simulink model "craig_control"  (R2016a)
settings: Solver=VariableStepAuto  StartTime=0.0  StopTime=tray_time  FixedStep=time_per_step  MaxStep=0.005  RelTol=1e-3
undefined symbols (not defined in the file): jacob0, kp, kv, my_inv_j, robot_model
libraries: roblocks x5, vector_sweep x2
settings Model: ExtModeTrigMode=oneshot  ExtModeArmWhenConnect=off  Creator=pic  LastModifiedBy=Nahuel
settings SolverCC: ZeroCrossControl=DisableAll
settings DataIOCC: SaveFormat=Array  SignalLoggingSaveFormat=ModelDataLogs  ReturnWorkspaceOutputs=on
settings OptimizationCC: BlockReduction=off  BooleanDataType=off  ExpressionDepthLimit=2147483647  InitFltsAndDblsToZero=on
settings DebuggingCC: SaveWithParameterizedLinksMsg=none  UnderspecifiedInitializationDetection=Classic  MergeDetectMultiDrivingBlocksExec=none  SignalResolutionControl=TryResolveAllWithWarning  MultiTaskDSMMsg=warning  MultiTaskCondExecSysMsg=none  FcnCallInpInsideContextMsg=UseLocalSettings  StateNameClashWarn=warning
settings HardwareCC: ProdBitPerPointer=32  ProdLargestAtomicFloat=None  ProdIntDivRoundTo=Undefined  ProdEndianess=Unspecified  ProdWordSize=32  ProdHWDeviceType=32-bit Generic  TargetUnknown=on
settings ModelReferenceCC: PropagateSignalLabelsOutOfModel=off
settings GRTTargetCC: ModelReferenceCompliant=off  CompOptLevelCompliant=off  CombineOutputUpdateFcns=off  MatFileLogging=off  GRTInterface=on
settings ConfigComp: CovModelRefEnable=Off

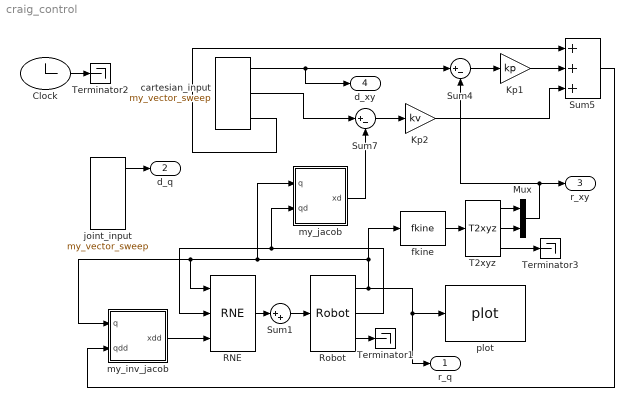
== system craig_control ==
  Clock : Clock
  Kp1 : Gain  Gain=kp  SaturateOnIntegerOverflow=on  OutDataTypeStr=Inherit: Same as input  ParamDataTypeStr=Inherit: Same as input
  Kp2 : Gain  Gain=kv  SaturateOnIntegerOverflow=on  OutDataTypeStr=Inherit: Same as input  ParamDataTypeStr=Inherit: Same as input
  Mux : Mux  Inputs=2
  RNE : roblocks/Dynamics/RNE  robot=robot_model  grav=[0 0 9.81]
  Robot : roblocks/Dynamics/Robot  robot=robot_real  q0=[-pi/2 pi/2]
  Sum1 : Sum  Inputs=|++  SaturateOnIntegerOverflow=on  InputSameDT=on  OutDataTypeStr=Inherit: Same as first input
  Sum4 : Sum  Inputs=|+-  SaturateOnIntegerOverflow=on  InputSameDT=on  OutDataTypeStr=Inherit: Same as first input
  Sum5 : Sum  Inputs=+++  SaturateOnIntegerOverflow=on  InputSameDT=on  OutDataTypeStr=Inherit: Same as first input
  Sum7 : Sum  Inputs=|+-  SaturateOnIntegerOverflow=on  InputSameDT=on  OutDataTypeStr=Inherit: Same as first input
  T2xyz : roblocks/Transform Conversion/T2xyz
  Terminator1 : Terminator
  Terminator2 : Terminator
  Terminator3 : Terminator
  cartesian_input : vector_sweep/my_vector_sweep  q_in=x_in  qd_in=xd_in  qdd_in=qdd_in  tmax=tray_time
  fkine : roblocks/Kinematics/fkine  robot=robot_model
  joint_input : vector_sweep/my_vector_sweep  q_in=q_in  qd_in=qd_in  qdd_in=qdd_in  tmax=tray_time
  my_inv_jacob : Subsystem  AncestorBlock=vector_sweep/my_inv_jacob
      mask help: Inverse Jacobian
      mask Help:
      | Inverse of Jacobian matrix which maps spatial velocity to joint coordinate
      | rates.
      | 
      | 
      | <b>Inputs::</b>
      | 
      | J (6x6) the Jacobian matrix
      | 
      | <b>Outputs::</b>
      | 
      | Ji (6x6) the inverse Jacobian matrix
      | 
      | <b>Notes::</b>
      | 
      | - A wrapper for the MATLAB function inv().
      | - Only valid for square Jacobians (6-axis robots)
      mask Display:
      | text(0.4, 0.7, '\bf\fontsize{16}J', 'texmode', 'on', 'verticalAlignment', 'top', 'horizontalAlignment', 'left')
      | text(0.6, 0.65, '\fontsize{10}-1', 'texmode', 'on','verticalAlignment', 'bottom', 'horizontalAlignment', 'left')
      | port_label('input', 1, 'q');
      | port_label('input', 2, 'xdd');
      | port_label('output', 1, 'qdd');
  "my_jacob " : Subsystem  AncestorBlock=vector_sweep/my_jacob  mask{robot=robot_model}
      mask prompts: robot "Robot object"
      mask help: Robot Jacobian in world coordinates
      mask init:
      | n=robot.n;
      mask Help:
      | Jacobian matrix relating joint coordinate rates to end-effector spatial
      | velocity expressed in the world frame.
      | 
      | <b>Parameters::</b>
      | 
      | Robot (SerialLink class)  The N-axis robot object for which the Jacobian is
      |                           computed.
      | 
      | <b>Inputs::</b>
      | 
      | q (1xN) joint coordinates
      | 
      | <b>Outputs::</b>
      | 
      | J (6xN) the Jacobian matrix
      | 
      | <b>Notes::</b>
      | 
      | - A wrapper for the Toolbox method jacob0().
      mask Display:
      | text(0.4, 0.7, '\bf\fontsize{16}J', 'texmode', 'on', 'verticalAlignment', 'top', 'horizontalAlignment', 'left')
      | text(0.45, 0.65, '\fontsize{10}0', 'texmode', 'on','verticalAlignment', 'bottom', 'horizontalAlignment', 'right')
      | if ~isempty(robot)
      |     text(0.5, 0.2, robot.name,  'horizontalAlignment', 'center')
      | end
      | port_label('input', 1, 'q')
      | port_label('input', 2, 'qd')
      | port_label('output', 1, 'xd')
  plot : roblocks/Robot Graphics/plot  robot=robot_real  fps=10  holdplot=on
  r_q : Outport
  d_q : Outport  Port=2
  r_xy : Outport  Port=3
  d_xy : Outport  Port=4
  wires:
  joint_input/1 -> d_q/1
  Robot/3 -> Terminator1/1
  Clock/1 -> Terminator2/1
  Robot/2 -> RNE/2, "my_jacob "/2(qd)
  fkine/1 -> T2xyz/1
  T2xyz/1 -> Mux/1
  T2xyz/2 -> Mux/2
  Robot/1 -> fkine/1, RNE/1, my_inv_jacob/1(q), "my_jacob "/1(q), plot/1, r_q/1
  cartesian_input/1 -> d_xy/1, Sum4/1
  Sum4/1 -> Kp1/1
  Kp1/1 -> Sum5/2
  cartesian_input/3 -> Sum5/1
  Kp2/1 -> Sum5/3
  Sum5/1 -> my_inv_jacob/2("qdd ")
  Sum7/1 -> Kp2/1
  "my_jacob "/1(xd) -> Sum7/2
  cartesian_input/2 -> Sum7/1
  Mux/1 -> Sum4/2, r_xy/1
  T2xyz/3 -> Terminator3/1
  my_inv_jacob/1(xdd) -> RNE/3
  Sum1/1 -> Robot/1
  RNE/1 -> Sum1/1

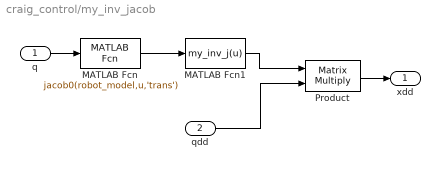
== system craig_control/my_inv_jacob ==
  q : Inport
  "qdd " : Inport  Port=2
  MATLAB Fcn : MATLABFcn  MATLABFcn=jacob0(robot_model,u,'trans')  OutputDimensions=[3 2]  Output1D=off
  MATLAB Fcn1 : MATLABFcn  MATLABFcn=my_inv_j(u)  OutputDimensions=[2 2]  Output1D=off
  Product : Product  Multiplication=Matrix(*)
  xdd : Outport
  wires:
  "qdd "/1 -> Product/2
  MATLAB Fcn1/1 -> Product/1
  MATLAB Fcn/1 -> MATLAB Fcn1/1
  Product/1 -> xdd/1
  q/1 -> MATLAB Fcn/1

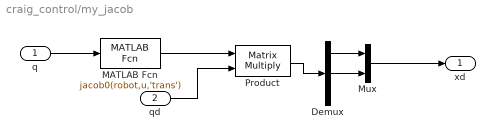
== system craig_control/my_jacob  ==
  q : Inport
  qd : Inport  Port=2
  Demux : Demux  Outputs=3
  MATLAB Fcn : MATLABFcn  MATLABFcn=jacob0(robot,u,'trans')  Output1D=off
  Mux : Mux  Inputs=2
  Product : Product  Multiplication=Matrix(*)
  xd : Outport
  wires:
  Product/1 -> Demux/1
  qd/1 -> Product/2
  q/1 -> MATLAB Fcn/1
  MATLAB Fcn/1 -> Product/1
  Demux/2 -> Mux/2
  Demux/1 -> Mux/1
  Mux/1 -> xd/1
